simulink subsystem "rocket_flight"  (R2025b)
settings: Solver=VariableStepAuto  StartTime=0.0  StopTime=10.0  RelTol=1e-3
undefined symbols (not defined in the file): I_xx, I_yy, location, mass, OR_cg, rail_angle_pitch, rail_angle_roll, rail_angle_yaw, sim_time, time_idle
libraries: matrix_library x2, aerolib6dof2 x1
settings Model: Creator=joedo  LastModifiedBy=finnb

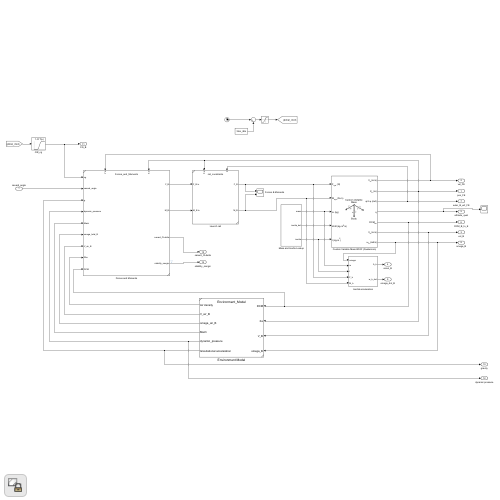
[thumbnail: Simulink's stored preview of the top-level diagram]
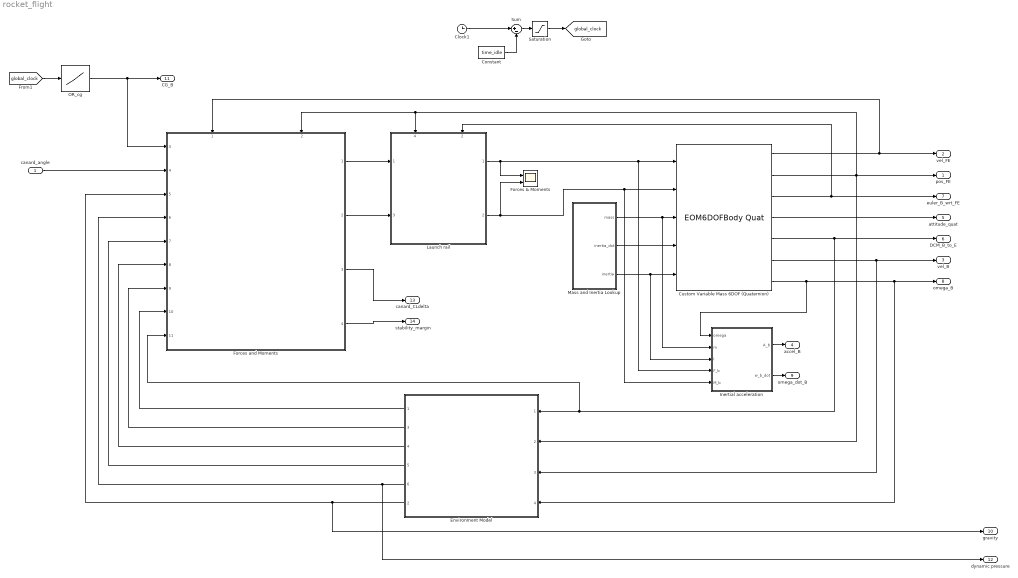
== system rocket_flight ==
  canard_angle : Inport
  Clock1 : Clock
  Constant : Constant  Value=time_idle
  Custom Variable Mass 6DOF (Quaternion) : EOM6DOFBodyQuat  mtype=Custom Variable  xme_0=[location(1) 0 0]  eul_0=[rail_angle_roll, rail_angle_pitch, rail_angle_yaw]
  Environment Model : Subsystem  ReferencedSubsystem=Environment_Model
      settings: PortSchema="{\"entries\":[{\"content\":{\"sides\":[{\"content\":{\"connectorIds\":[\"In1\",\"In2\",\"In3\",\"In4\"]},\"type\":\"ConnectorPlacement.EquallySpacedRectSide\",\"uuid\":\"2a81b9c5-b150-4b95-94af-394a03d0678a\"},{\"content\":{\"connectorIds\":[\"Out1\",\"Out3\",\"Out4\",\"Out5\",\"Out6\",\"Out2\"],\"side\":\"RIGHT\"},\"type\":\"ConnectorPlacement.EquallySpacedRectSide\",\"uuid\":\"876dc6e2-e5c6-4258-adc0-40f09f61a15a\"},{\"content\":{\"side\":\"TOP\"},\"type\":\"ConnectorPlacement.EquallySpacedRectSide\",\"uuid\":\"30ca8b3b-9b10-4b0a-a581-f2563a0e4844\"}]},\"type\":\"ConnectorPlacement.EquallySpacedConnector\",\"uuid\":\"0a44bd71-bf6b-4260-a474-a2581db635e7\"}],\"packageUris\":[\"http://schema.mathworks.com/mf0/Connector/R2020b\"],\"version\":\"1.0\"}"
  Forces & Moments : Scope  NumInputPorts=2
      settings: ActiveDisplayYMinimum=-1694.65546  ActiveDisplayYMaximum=8529.99885
  "Forces and Moments " : Subsystem  ReferencedSubsystem=Forces_and_Moments
      settings: PortSchema="{\"entries\":[{\"content\":{\"sides\":[{\"content\":{\"connectorIds\":[\"In3\",\"In4\",\"In5\",\"In6\",\"In7\",\"In8\",\"In9\",\"In10\",\"In11\"]},\"type\":\"ConnectorPlacement.EquallySpacedRectSide\",\"uuid\":\"2d9b15f2-fc7e-4399-b4ca-f7faa58838df\"},{\"content\":{\"connectorIds\":[\"Out1\",\"Out2\",\"Out3\",\"Out4\"],\"side\":\"RIGHT\"},\"type\":\"ConnectorPlacement.EquallySpacedRectSide\",\"uuid\":\"cd9b89d4-ce85-488b-9a3f-64297ccf9b96\"},{\"content\":{\"connectorIds\":[\"In1\",\"In2\"],\"side\":\"TOP\"},\"type\":\"ConnectorPlacement.EquallySpacedRectSide\",\"uuid\":\"472a10a7-0072-45c6-a8aa-5eaf234894da\"}]},\"type\":\"ConnectorPlacement.EquallySpacedConnector\",\"uuid\":\"79d150c0-9861-42cf-8cdc-8f9e609deb28\"}],\"packageUris\":[\"http://schema.mathworks.com/mf0/Connector/R2020b\"],\"version\":\"1.0\"}"
  Inertial acceleration : Subsystem
  Launch rail : Subsystem  ReferencedSubsystem=rail_constraints
      settings: PortSchema="{\"entries\":[{\"content\":{\"sides\":[{\"content\":{\"connectorIds\":[\"In1\",\"In3\"]},\"type\":\"ConnectorPlacement.EquallySpacedRectSide\",\"uuid\":\"f8bc89cf-4366-4095-a699-e573bc22001a\"},{\"content\":{\"connectorIds\":[\"Out1\",\"Out2\"],\"side\":\"RIGHT\"},\"type\":\"ConnectorPlacement.EquallySpacedRectSide\",\"uuid\":\"f55d6fa0-3d5e-48fa-b07b-9e72276225fb\"},{\"content\":{\"connectorIds\":[\"In4\",\"In2\"],\"side\":\"TOP\"},\"type\":\"ConnectorPlacement.EquallySpacedRectSide\",\"uuid\":\"5696589c-23a4-46a9-b349-1864b914459a\"}]},\"type\":\"ConnectorPlacement.EquallySpacedConnector\",\"uuid\":\"1b8f695c-cf97-4880-abd1-8dadf97d6ecb\"}],\"packageUris\":[\"http://schema.mathworks.com/mf0/Connector/R2020b\"],\"version\":\"1.0\"}"
  Mass and Inertia Lookup : Subsystem
  OR_cg : Lookup_n-D  NumberOfTableDimensions=1  BreakpointsForDimension1=sim_time  Table=OR_cg  InternalRulePriority=Speed  RndMeth=Simplest
  Saturation : Saturate  UpperLimit=inf  LowerLimit=0
  Sum : Sum  Inputs=|+-
  pos_FE : Outport
  vel_FE : Outport  Port=2
  vel_B : Outport  Port=3  PortDimensions=3
  accel_B : Outport  Port=4  PortDimensions=3
  attitude_quat : Outport  Port=5
  DCM_B_to_E : Outport  Port=6
  euler_B_wrt_FE : Outport  Port=7
  omega_B : Outport  Port=8
  omega_dot_B : Outport  Port=9
  gravity : Outport  Port=10
  CG_B : Outport  Port=11
  dynamic pressure : Outport  Port=12
  canard_CLdelta : Outport  Port=13
  stability_margin : Outport  Port=14
  tag scope: global_clock=global
  wires:
  Custom Variable Mass 6DOF (Quaternion)/7 -> Environment Model/4, omega_B/1, Inertial acceleration/1(omega)
  "Forces and Moments "/2 -> Launch rail/3
  Launch rail/2 -> Inertial acceleration/5(M_b), Custom Variable Mass 6DOF (Quaternion)/2, Forces & Moments/2
  "Forces and Moments "/4 -> stability_margin/1
  "Forces and Moments "/3 -> canard_CLdelta/1
  "Forces and Moments "/1 -> Launch rail/1
  Environment Model/6 -> "Forces and Moments "/6, dynamic pressure/1
  Environment Model/3 -> "Forces and Moments "/9
  Custom Variable Mass 6DOF (Quaternion)/4 -> attitude_quat/1
  Saturation/1 -> [global_clock]
  Constant/1 -> Sum/2
  Sum/1 -> Saturation/1
  Clock1/1 -> Sum/1
  OR_cg/1 -> CG_B/1, "Forces and Moments "/3
  [global_clock] -> OR_cg/1
  Custom Variable Mass 6DOF (Quaternion)/5 -> "Forces and Moments "/11, Environment Model/1, DCM_B_to_E/1
  Custom Variable Mass 6DOF (Quaternion)/3 -> euler_B_wrt_FE/1, Launch rail/2
  Custom Variable Mass 6DOF (Quaternion)/1 -> vel_FE/1, "Forces and Moments "/1
  Environment Model/2 -> gravity/1, "Forces and Moments "/5
  Environment Model/5 -> "Forces and Moments "/7
  Custom Variable Mass 6DOF (Quaternion)/2 -> Environment Model/2, pos_FE/1, "Forces and Moments "/2, Launch rail/4
  Environment Model/1 -> "Forces and Moments "/10
  Environment Model/4 -> "Forces and Moments "/8
  Custom Variable Mass 6DOF (Quaternion)/6 -> Environment Model/3, vel_B/1
  canard_angle/1 -> "Forces and Moments "/4
  Mass and Inertia Lookup/1(mass) -> Inertial acceleration/2(m), Custom Variable Mass 6DOF (Quaternion)/3
  Launch rail/1 -> Forces & Moments/1, Inertial acceleration/4(F_b), Custom Variable Mass 6DOF (Quaternion)/1
  Inertial acceleration/1(A_b) -> accel_B/1
  Inertial acceleration/2(w_b_dot) -> omega_dot_B/1
  Mass and Inertia Lookup/2(inertia_dot) -> Custom Variable Mass 6DOF (Quaternion)/4
  Mass and Inertia Lookup/3(inertia) -> Custom Variable Mass 6DOF (Quaternion)/5, Inertial acceleration/3(I)

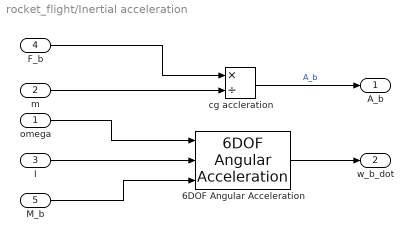
== system rocket_flight/Inertial acceleration ==
  omega : Inport
  m : Inport  Port=2
  I : Inport  Port=3
  F_b : Inport  Port=4
  M_b : Inport  Port=5
  6DOF Angular Acceleration : aerolib6dof2/6DOF Angular Acceleration  units=Metric (MKS)  mtype=Fixed
  cg accleration : Product  Inputs=*/
  A_b : Outport
  w_b_dot : Outport  Port=2
  wires:
  F_b/1 -> cg accleration/1
  M_b/1 -> 6DOF Angular Acceleration/3
  m/1 -> cg accleration/2
  6DOF Angular Acceleration/1 -> w_b_dot/1
  I/1 -> 6DOF Angular Acceleration/2
  omega/1 -> 6DOF Angular Acceleration/1
  cg accleration/1 -> A_b/1  "A_b"

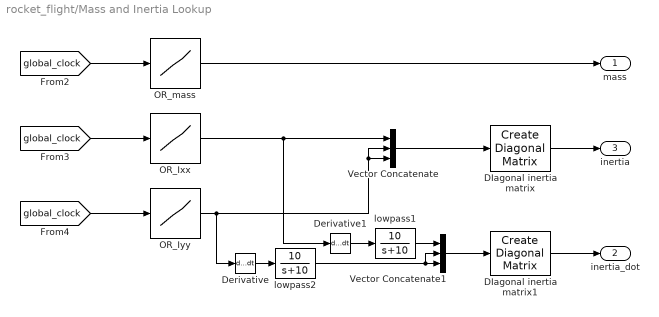
== system rocket_flight/Mass and Inertia Lookup ==
  DIagonal inertia matrix : matrix_library/Create Diagonal Matrix
      settings: LibrarySourceBlock=|
      | simulink/Matrix
      | Operations/Create Diagonal
      | Matrix
  DIagonal inertia matrix1 : matrix_library/Create Diagonal Matrix
      settings: LibrarySourceBlock=|
      | simulink/Matrix
      | Operations/Create Diagonal
      | Matrix
  Derivative : Derivative
  Derivative1 : Derivative
  OR_Ixx : Lookup_n-D  NumberOfTableDimensions=1  BreakpointsForDimension1=sim_time  Table=I_xx  InternalRulePriority=Speed  RndMeth=Simplest
  OR_Iyy : Lookup_n-D  NumberOfTableDimensions=1  BreakpointsForDimension1=sim_time  Table=I_yy  InternalRulePriority=Speed  RndMeth=Simplest
  OR_mass : Lookup_n-D  NumberOfTableDimensions=1  BreakpointsForDimension1=sim_time  Table=mass  InternalRulePriority=Speed  RndMeth=Simplest
  Vector Concatenate : Concatenate  NumInputs=3
  Vector Concatenate1 : Concatenate  NumInputs=3
  lowpass1 : TransferFcn  Numerator=[10]  Denominator=[1 10]
  lowpass2 : TransferFcn  Numerator=[10]  Denominator=[1 10]
  mass : Outport
  inertia_dot : Outport  Port=2
  inertia : Outport  Port=3
  wires:
  lowpass2/1 -> Vector Concatenate1/2, Vector Concatenate1/3
  lowpass1/1 -> Vector Concatenate1/1
  Derivative1/1 -> lowpass1/1
  Derivative/1 -> lowpass2/1
  DIagonal inertia matrix1/1 -> inertia_dot/1
  Vector Concatenate/1 -> DIagonal inertia matrix/1
  [global_clock] -> OR_mass/1
  Vector Concatenate1/1 -> DIagonal inertia matrix1/1
  [global_clock] -> OR_Ixx/1
  [global_clock] -> OR_Iyy/1
  OR_Ixx/1 -> Vector Concatenate/1, Derivative1/1
  DIagonal inertia matrix/1 -> inertia/1
  OR_mass/1 -> mass/1
  OR_Iyy/1 -> Vector Concatenate/3, Vector Concatenate/2, Derivative/1
